simulink model "elevator"  (R2020a)
settings: Solver=VariableStepAuto  StartTime=0.0  StopTime=inf  RelTol=1e-3
PreLoadFcn:
  | slplc.api.loadDataTypes;
undefined symbols (not defined in the file): BOOL, DINT, INT, slplc
libraries: simulink x1
(part 10 of 38)

== system elevator/PLCControllerSuite/__Logic/Task/Program/__Logic/XIC60 ==
  RungIn : Inport  PortDimensions=1
  BlockEnableRead : Subsystem  DisableCoverage=on  TreatAsAtomicUnit=on  mask{PLCLabelTag=_Block_Enable, PLCBlockType=BlockEnableRead}
      mask prompts: PLCLabelTag "Label Tag:"
      mask init:
      | block = gcb;
      | maskObj = Simulink.Mask.get(block);
      | maskObj.Display = sprintf('disp(''%s'');', PLCLabelTag);
      mask Help: web([docroot '/plccoder/ref/blockenableread' '.html']);
      mask DialogControl PLCBlockTitle Prompt: Block Enable Read
      mask Display: disp('_Block_Enable');
  Instruction_Enable : Subsystem  Priority=12  TreatAsAtomicUnit=on
  RungInOverride : Subsystem  DisableCoverage=on  TreatAsAtomicUnit=on
  __CoreVarRead : Subsystem  Tag=CoreVarReadBlock  DisableCoverage=on  TreatAsAtomicUnit=on  mask{PLCBlockType=CoreVarRead}
      mask init:
      | slplc.callbacks.initCoreVariable(gcb, 'read');
      mask Help: web([docroot '/plccoder/ref/__corevarread' '.html']);
      mask DialogControl PLCBlockTitle Prompt: Core Variable Read
  __Format : MATLAB Function  Tag=PLC_Format_Boolean  Priority=20  DisableCoverage=on  InitFcn=slplc.utils.setBlockAppearance('reset', '%<PLCOperandTag>');  StopFcn=slplc.utils.setBlockAppearance('reset', '%<PLCOperandTag>');  TreatAsAtomicUnit=on
  RungOut : Outport  OutDataTypeStr=BOOL  PortDimensions=1  InitialOutput=false  VectorParamsAs1DForOutWhenUnconnected=off
  wires:
  RungIn/1 -> RungInOverride/1(In1)
  Instruction_Enable/1(Rung-condition-out) -> __Format/3(RungOut), RungOut/1
  BlockEnableRead/1(Out1) -> __Format/1(BlockEnable), Instruction_Enable/Enable
  RungInOverride/1(Out1) -> __Format/2(RungIn), Instruction_Enable/1(Rung-condition-in)
  __CoreVarRead/1(y) -> __Format/4(data)  "DataBit"

== system elevator/PLCControllerSuite/__Logic/Task/Program/__Logic/XIC61 ==
  RungIn : Inport  PortDimensions=1
  BlockEnableRead : Subsystem  DisableCoverage=on  TreatAsAtomicUnit=on  mask{PLCLabelTag=_Block_Enable, PLCBlockType=BlockEnableRead}
      mask prompts: PLCLabelTag "Label Tag:"
      mask init:
      | block = gcb;
      | maskObj = Simulink.Mask.get(block);
      | maskObj.Display = sprintf('disp(''%s'');', PLCLabelTag);
      mask Help: web([docroot '/plccoder/ref/blockenableread' '.html']);
      mask DialogControl PLCBlockTitle Prompt: Block Enable Read
      mask Display: disp('_Block_Enable');
  Instruction_Enable : Subsystem  Priority=12  TreatAsAtomicUnit=on
  RungInOverride : Subsystem  DisableCoverage=on  TreatAsAtomicUnit=on
  __CoreVarRead : Subsystem  Tag=CoreVarReadBlock  DisableCoverage=on  TreatAsAtomicUnit=on  mask{PLCBlockType=CoreVarRead}
      mask init:
      | slplc.callbacks.initCoreVariable(gcb, 'read');
      mask Help: web([docroot '/plccoder/ref/__corevarread' '.html']);
      mask DialogControl PLCBlockTitle Prompt: Core Variable Read
  __Format : MATLAB Function  Tag=PLC_Format_Boolean  Priority=20  DisableCoverage=on  InitFcn=slplc.utils.setBlockAppearance('reset', '%<PLCOperandTag>');  StopFcn=slplc.utils.setBlockAppearance('reset', '%<PLCOperandTag>');  TreatAsAtomicUnit=on
  RungOut : Outport  OutDataTypeStr=BOOL  PortDimensions=1  InitialOutput=false  VectorParamsAs1DForOutWhenUnconnected=off
  wires:
  __CoreVarRead/1(y) -> __Format/4(data)  "DataBit"
  RungInOverride/1(Out1) -> Instruction_Enable/1(Rung-condition-in), __Format/2(RungIn)
  BlockEnableRead/1(Out1) -> Instruction_Enable/Enable, __Format/1(BlockEnable)
  Instruction_Enable/1(Rung-condition-out) -> RungOut/1, __Format/3(RungOut)
  RungIn/1 -> RungInOverride/1(In1)

== system elevator/PLCControllerSuite/__Logic/Task/Program/__Logic/XIC62 ==
  RungIn : Inport  PortDimensions=1
  BlockEnableRead : Subsystem  DisableCoverage=on  TreatAsAtomicUnit=on  mask{PLCLabelTag=_Block_Enable, PLCBlockType=BlockEnableRead}
      mask prompts: PLCLabelTag "Label Tag:"
      mask init:
      | block = gcb;
      | maskObj = Simulink.Mask.get(block);
      | maskObj.Display = sprintf('disp(''%s'');', PLCLabelTag);
      mask Help: web([docroot '/plccoder/ref/blockenableread' '.html']);
      mask DialogControl PLCBlockTitle Prompt: Block Enable Read
      mask Display: disp('_Block_Enable');
  Instruction_Enable : Subsystem  Priority=12  TreatAsAtomicUnit=on
  RungInOverride : Subsystem  DisableCoverage=on  TreatAsAtomicUnit=on
  __CoreVarRead : Subsystem  Tag=CoreVarReadBlock  DisableCoverage=on  TreatAsAtomicUnit=on  mask{PLCBlockType=CoreVarRead}
      mask init:
      | slplc.callbacks.initCoreVariable(gcb, 'read');
      mask Help: web([docroot '/plccoder/ref/__corevarread' '.html']);
      mask DialogControl PLCBlockTitle Prompt: Core Variable Read
  __Format : MATLAB Function  Tag=PLC_Format_Boolean  Priority=20  DisableCoverage=on  InitFcn=slplc.utils.setBlockAppearance('reset', '%<PLCOperandTag>');  StopFcn=slplc.utils.setBlockAppearance('reset', '%<PLCOperandTag>');  TreatAsAtomicUnit=on
  RungOut : Outport  OutDataTypeStr=BOOL  PortDimensions=1  InitialOutput=false  VectorParamsAs1DForOutWhenUnconnected=off
  wires:
  __CoreVarRead/1(y) -> __Format/4(data)  "DataBit"
  RungInOverride/1(Out1) -> Instruction_Enable/1(Rung-condition-in), __Format/2(RungIn)
  BlockEnableRead/1(Out1) -> Instruction_Enable/Enable, __Format/1(BlockEnable)
  Instruction_Enable/1(Rung-condition-out) -> RungOut/1, __Format/3(RungOut)
  RungIn/1 -> RungInOverride/1(In1)

== system elevator/PLCControllerSuite/__Logic/Task/Program/__Logic/XIC63 ==
  RungIn : Inport  PortDimensions=1
  BlockEnableRead : Subsystem  DisableCoverage=on  TreatAsAtomicUnit=on  mask{PLCLabelTag=_Block_Enable, PLCBlockType=BlockEnableRead}
      mask prompts: PLCLabelTag "Label Tag:"
      mask init:
      | block = gcb;
      | maskObj = Simulink.Mask.get(block);
      | maskObj.Display = sprintf('disp(''%s'');', PLCLabelTag);
      mask Help: web([docroot '/plccoder/ref/blockenableread' '.html']);
      mask DialogControl PLCBlockTitle Prompt: Block Enable Read
      mask Display: disp('_Block_Enable');
  Instruction_Enable : Subsystem  Priority=12  TreatAsAtomicUnit=on
  RungInOverride : Subsystem  DisableCoverage=on  TreatAsAtomicUnit=on
  __CoreVarRead : Subsystem  Tag=CoreVarReadBlock  DisableCoverage=on  TreatAsAtomicUnit=on  mask{PLCBlockType=CoreVarRead}
      mask init:
      | slplc.callbacks.initCoreVariable(gcb, 'read');
      mask Help: web([docroot '/plccoder/ref/__corevarread' '.html']);
      mask DialogControl PLCBlockTitle Prompt: Core Variable Read
  __Format : MATLAB Function  Tag=PLC_Format_Boolean  Priority=20  DisableCoverage=on  InitFcn=slplc.utils.setBlockAppearance('reset', '%<PLCOperandTag>');  StopFcn=slplc.utils.setBlockAppearance('reset', '%<PLCOperandTag>');  TreatAsAtomicUnit=on
  RungOut : Outport  OutDataTypeStr=BOOL  PortDimensions=1  InitialOutput=false  VectorParamsAs1DForOutWhenUnconnected=off
  wires:
  RungIn/1 -> RungInOverride/1(In1)
  Instruction_Enable/1(Rung-condition-out) -> __Format/3(RungOut), RungOut/1
  BlockEnableRead/1(Out1) -> __Format/1(BlockEnable), Instruction_Enable/Enable
  RungInOverride/1(Out1) -> __Format/2(RungIn), Instruction_Enable/1(Rung-condition-in)
  __CoreVarRead/1(y) -> __Format/4(data)  "DataBit"

== system elevator/PLCControllerSuite/__Logic/Task/Program/__Logic/XIC64 ==
  RungIn : Inport  PortDimensions=1
  BlockEnableRead : Subsystem  DisableCoverage=on  TreatAsAtomicUnit=on  mask{PLCLabelTag=_Block_Enable, PLCBlockType=BlockEnableRead}
      mask prompts: PLCLabelTag "Label Tag:"
      mask init:
      | block = gcb;
      | maskObj = Simulink.Mask.get(block);
      | maskObj.Display = sprintf('disp(''%s'');', PLCLabelTag);
      mask Help: web([docroot '/plccoder/ref/blockenableread' '.html']);
      mask DialogControl PLCBlockTitle Prompt: Block Enable Read
      mask Display: disp('_Block_Enable');
  Instruction_Enable : Subsystem  Priority=12  TreatAsAtomicUnit=on
  RungInOverride : Subsystem  DisableCoverage=on  TreatAsAtomicUnit=on
  __CoreVarRead : Subsystem  Tag=CoreVarReadBlock  DisableCoverage=on  TreatAsAtomicUnit=on  mask{PLCBlockType=CoreVarRead}
      mask init:
      | slplc.callbacks.initCoreVariable(gcb, 'read');
      mask Help: web([docroot '/plccoder/ref/__corevarread' '.html']);
      mask DialogControl PLCBlockTitle Prompt: Core Variable Read
  __Format : MATLAB Function  Tag=PLC_Format_Boolean  Priority=20  DisableCoverage=on  InitFcn=slplc.utils.setBlockAppearance('reset', '%<PLCOperandTag>');  StopFcn=slplc.utils.setBlockAppearance('reset', '%<PLCOperandTag>');  TreatAsAtomicUnit=on
  RungOut : Outport  OutDataTypeStr=BOOL  PortDimensions=1  InitialOutput=false  VectorParamsAs1DForOutWhenUnconnected=off
  wires:
  RungIn/1 -> RungInOverride/1(In1)
  Instruction_Enable/1(Rung-condition-out) -> __Format/3(RungOut), RungOut/1
  BlockEnableRead/1(Out1) -> __Format/1(BlockEnable), Instruction_Enable/Enable
  RungInOverride/1(Out1) -> __Format/2(RungIn), Instruction_Enable/1(Rung-condition-in)
  __CoreVarRead/1(y) -> __Format/4(data)  "DataBit"

== system elevator/PLCControllerSuite/__Logic/Task/Program/__Logic/XIC65 ==
  RungIn : Inport  PortDimensions=1
  BlockEnableRead : Subsystem  DisableCoverage=on  TreatAsAtomicUnit=on  mask{PLCLabelTag=_Block_Enable, PLCBlockType=BlockEnableRead}
      mask prompts: PLCLabelTag "Label Tag:"
      mask init:
      | block = gcb;
      | maskObj = Simulink.Mask.get(block);
      | maskObj.Display = sprintf('disp(''%s'');', PLCLabelTag);
      mask Help: web([docroot '/plccoder/ref/blockenableread' '.html']);
      mask DialogControl PLCBlockTitle Prompt: Block Enable Read
      mask Display: disp('_Block_Enable');
  Instruction_Enable : Subsystem  Priority=12  TreatAsAtomicUnit=on
  RungInOverride : Subsystem  DisableCoverage=on  TreatAsAtomicUnit=on
  __CoreVarRead : Subsystem  Tag=CoreVarReadBlock  DisableCoverage=on  TreatAsAtomicUnit=on  mask{PLCBlockType=CoreVarRead}
      mask init:
      | slplc.callbacks.initCoreVariable(gcb, 'read');
      mask Help: web([docroot '/plccoder/ref/__corevarread' '.html']);
      mask DialogControl PLCBlockTitle Prompt: Core Variable Read
  __Format : MATLAB Function  Tag=PLC_Format_Boolean  Priority=20  DisableCoverage=on  InitFcn=slplc.utils.setBlockAppearance('reset', '%<PLCOperandTag>');  StopFcn=slplc.utils.setBlockAppearance('reset', '%<PLCOperandTag>');  TreatAsAtomicUnit=on
  RungOut : Outport  OutDataTypeStr=BOOL  PortDimensions=1  InitialOutput=false  VectorParamsAs1DForOutWhenUnconnected=off
  wires:
  __CoreVarRead/1(y) -> __Format/4(data)  "DataBit"
  RungInOverride/1(Out1) -> Instruction_Enable/1(Rung-condition-in), __Format/2(RungIn)
  BlockEnableRead/1(Out1) -> Instruction_Enable/Enable, __Format/1(BlockEnable)
  Instruction_Enable/1(Rung-condition-out) -> RungOut/1, __Format/3(RungOut)
  RungIn/1 -> RungInOverride/1(In1)

== system elevator/PLCControllerSuite/__Logic/Task/Program/__Logic/XIC66 ==
  RungIn : Inport  PortDimensions=1
  BlockEnableRead : Subsystem  DisableCoverage=on  TreatAsAtomicUnit=on  mask{PLCLabelTag=_Block_Enable, PLCBlockType=BlockEnableRead}
      mask prompts: PLCLabelTag "Label Tag:"
      mask init:
      | block = gcb;
      | maskObj = Simulink.Mask.get(block);
      | maskObj.Display = sprintf('disp(''%s'');', PLCLabelTag);
      mask Help: web([docroot '/plccoder/ref/blockenableread' '.html']);
      mask DialogControl PLCBlockTitle Prompt: Block Enable Read
      mask Display: disp('_Block_Enable');
  Instruction_Enable : Subsystem  Priority=12  TreatAsAtomicUnit=on
  RungInOverride : Subsystem  DisableCoverage=on  TreatAsAtomicUnit=on
  __CoreVarRead : Subsystem  Tag=CoreVarReadBlock  DisableCoverage=on  TreatAsAtomicUnit=on  mask{PLCBlockType=CoreVarRead}
      mask init:
      | slplc.callbacks.initCoreVariable(gcb, 'read');
      mask Help: web([docroot '/plccoder/ref/__corevarread' '.html']);
      mask DialogControl PLCBlockTitle Prompt: Core Variable Read
  __Format : MATLAB Function  Tag=PLC_Format_Boolean  Priority=20  DisableCoverage=on  InitFcn=slplc.utils.setBlockAppearance('reset', '%<PLCOperandTag>');  StopFcn=slplc.utils.setBlockAppearance('reset', '%<PLCOperandTag>');  TreatAsAtomicUnit=on
  RungOut : Outport  OutDataTypeStr=BOOL  PortDimensions=1  InitialOutput=false  VectorParamsAs1DForOutWhenUnconnected=off
  wires:
  __CoreVarRead/1(y) -> __Format/4(data)  "DataBit"
  RungInOverride/1(Out1) -> Instruction_Enable/1(Rung-condition-in), __Format/2(RungIn)
  BlockEnableRead/1(Out1) -> Instruction_Enable/Enable, __Format/1(BlockEnable)
  Instruction_Enable/1(Rung-condition-out) -> RungOut/1, __Format/3(RungOut)
  RungIn/1 -> RungInOverride/1(In1)

== system elevator/PLCControllerSuite/__Logic/Task/Program/__Logic/XIC67 ==
  RungIn : Inport  PortDimensions=1
  BlockEnableRead : Subsystem  DisableCoverage=on  TreatAsAtomicUnit=on  mask{PLCLabelTag=_Block_Enable, PLCBlockType=BlockEnableRead}
      mask prompts: PLCLabelTag "Label Tag:"
      mask init:
      | block = gcb;
      | maskObj = Simulink.Mask.get(block);
      | maskObj.Display = sprintf('disp(''%s'');', PLCLabelTag);
      mask Help: web([docroot '/plccoder/ref/blockenableread' '.html']);
      mask DialogControl PLCBlockTitle Prompt: Block Enable Read
      mask Display: disp('_Block_Enable');
  Instruction_Enable : Subsystem  Priority=12  TreatAsAtomicUnit=on
  RungInOverride : Subsystem  DisableCoverage=on  TreatAsAtomicUnit=on
  __CoreVarRead : Subsystem  Tag=CoreVarReadBlock  DisableCoverage=on  TreatAsAtomicUnit=on  mask{PLCBlockType=CoreVarRead}
      mask init:
      | slplc.callbacks.initCoreVariable(gcb, 'read');
      mask Help: web([docroot '/plccoder/ref/__corevarread' '.html']);
      mask DialogControl PLCBlockTitle Prompt: Core Variable Read
  __Format : MATLAB Function  Tag=PLC_Format_Boolean  Priority=20  DisableCoverage=on  InitFcn=slplc.utils.setBlockAppearance('reset', '%<PLCOperandTag>');  StopFcn=slplc.utils.setBlockAppearance('reset', '%<PLCOperandTag>');  TreatAsAtomicUnit=on
  RungOut : Outport  OutDataTypeStr=BOOL  PortDimensions=1  InitialOutput=false  VectorParamsAs1DForOutWhenUnconnected=off
  wires:
  RungIn/1 -> RungInOverride/1(In1)
  Instruction_Enable/1(Rung-condition-out) -> __Format/3(RungOut), RungOut/1
  BlockEnableRead/1(Out1) -> __Format/1(BlockEnable), Instruction_Enable/Enable
  RungInOverride/1(Out1) -> __Format/2(RungIn), Instruction_Enable/1(Rung-condition-in)
  __CoreVarRead/1(y) -> __Format/4(data)  "DataBit"

== system elevator/PLCControllerSuite/__Logic/Task/Program/__Logic/XIC68 ==
  RungIn : Inport  PortDimensions=1
  BlockEnableRead : Subsystem  DisableCoverage=on  TreatAsAtomicUnit=on  mask{PLCLabelTag=_Block_Enable, PLCBlockType=BlockEnableRead}
      mask prompts: PLCLabelTag "Label Tag:"
      mask init:
      | block = gcb;
      | maskObj = Simulink.Mask.get(block);
      | maskObj.Display = sprintf('disp(''%s'');', PLCLabelTag);
      mask Help: web([docroot '/plccoder/ref/blockenableread' '.html']);
      mask DialogControl PLCBlockTitle Prompt: Block Enable Read
      mask Display: disp('_Block_Enable');
  Instruction_Enable : Subsystem  Priority=12  TreatAsAtomicUnit=on
  RungInOverride : Subsystem  DisableCoverage=on  TreatAsAtomicUnit=on
  __CoreVarRead : Subsystem  Tag=CoreVarReadBlock  DisableCoverage=on  TreatAsAtomicUnit=on  mask{PLCBlockType=CoreVarRead}
      mask init:
      | slplc.callbacks.initCoreVariable(gcb, 'read');
      mask Help: web([docroot '/plccoder/ref/__corevarread' '.html']);
      mask DialogControl PLCBlockTitle Prompt: Core Variable Read
  __Format : MATLAB Function  Tag=PLC_Format_Boolean  Priority=20  DisableCoverage=on  InitFcn=slplc.utils.setBlockAppearance('reset', '%<PLCOperandTag>');  StopFcn=slplc.utils.setBlockAppearance('reset', '%<PLCOperandTag>');  TreatAsAtomicUnit=on
  RungOut : Outport  OutDataTypeStr=BOOL  PortDimensions=1  InitialOutput=false  VectorParamsAs1DForOutWhenUnconnected=off
  wires:
  __CoreVarRead/1(y) -> __Format/4(data)  "DataBit"
  RungInOverride/1(Out1) -> Instruction_Enable/1(Rung-condition-in), __Format/2(RungIn)
  BlockEnableRead/1(Out1) -> Instruction_Enable/Enable, __Format/1(BlockEnable)
  Instruction_Enable/1(Rung-condition-out) -> RungOut/1, __Format/3(RungOut)
  RungIn/1 -> RungInOverride/1(In1)

== system elevator/PLCControllerSuite/__Logic/Task/Program/__Logic/XIC69 ==
  RungIn : Inport  PortDimensions=1
  BlockEnableRead : Subsystem  DisableCoverage=on  TreatAsAtomicUnit=on  mask{PLCLabelTag=_Block_Enable, PLCBlockType=BlockEnableRead}
      mask prompts: PLCLabelTag "Label Tag:"
      mask init:
      | block = gcb;
      | maskObj = Simulink.Mask.get(block);
      | maskObj.Display = sprintf('disp(''%s'');', PLCLabelTag);
      mask Help: web([docroot '/plccoder/ref/blockenableread' '.html']);
      mask DialogControl PLCBlockTitle Prompt: Block Enable Read
      mask Display: disp('_Block_Enable');
  Instruction_Enable : Subsystem  Priority=12  TreatAsAtomicUnit=on
  RungInOverride : Subsystem  DisableCoverage=on  TreatAsAtomicUnit=on
  __CoreVarRead : Subsystem  Tag=CoreVarReadBlock  DisableCoverage=on  TreatAsAtomicUnit=on  mask{PLCBlockType=CoreVarRead}
      mask init:
      | slplc.callbacks.initCoreVariable(gcb, 'read');
      mask Help: web([docroot '/plccoder/ref/__corevarread' '.html']);
      mask DialogControl PLCBlockTitle Prompt: Core Variable Read
  __Format : MATLAB Function  Tag=PLC_Format_Boolean  Priority=20  DisableCoverage=on  InitFcn=slplc.utils.setBlockAppearance('reset', '%<PLCOperandTag>');  StopFcn=slplc.utils.setBlockAppearance('reset', '%<PLCOperandTag>');  TreatAsAtomicUnit=on
  RungOut : Outport  OutDataTypeStr=BOOL  PortDimensions=1  InitialOutput=false  VectorParamsAs1DForOutWhenUnconnected=off
  wires:
  RungIn/1 -> RungInOverride/1(In1)
  Instruction_Enable/1(Rung-condition-out) -> __Format/3(RungOut), RungOut/1
  BlockEnableRead/1(Out1) -> __Format/1(BlockEnable), Instruction_Enable/Enable
  RungInOverride/1(Out1) -> __Format/2(RungIn), Instruction_Enable/1(Rung-condition-in)
  __CoreVarRead/1(y) -> __Format/4(data)  "DataBit"

== system elevator/PLCControllerSuite/__Logic/Task/Program/__Logic/XIC7 ==
  RungIn : Inport  PortDimensions=1
  BlockEnableRead : Subsystem  DisableCoverage=on  TreatAsAtomicUnit=on  mask{PLCLabelTag=_Block_Enable, PLCBlockType=BlockEnableRead}
      mask prompts: PLCLabelTag "Label Tag:"
      mask init:
      | block = gcb;
      | maskObj = Simulink.Mask.get(block);
      | maskObj.Display = sprintf('disp(''%s'');', PLCLabelTag);
      mask Help: web([docroot '/plccoder/ref/blockenableread' '.html']);
      mask DialogControl PLCBlockTitle Prompt: Block Enable Read
      mask Display: disp('_Block_Enable');
  Instruction_Enable : Subsystem  Priority=12  TreatAsAtomicUnit=on
  RungInOverride : Subsystem  DisableCoverage=on  TreatAsAtomicUnit=on
  __CoreVarRead : Subsystem  Tag=CoreVarReadBlock  DisableCoverage=on  TreatAsAtomicUnit=on  mask{PLCBlockType=CoreVarRead}
      mask init:
      | slplc.callbacks.initCoreVariable(gcb, 'read');
      mask Help: web([docroot '/plccoder/ref/__corevarread' '.html']);
      mask DialogControl PLCBlockTitle Prompt: Core Variable Read
  __Format : MATLAB Function  Tag=PLC_Format_Boolean  Priority=20  DisableCoverage=on  InitFcn=slplc.utils.setBlockAppearance('reset', '%<PLCOperandTag>');  StopFcn=slplc.utils.setBlockAppearance('reset', '%<PLCOperandTag>');  TreatAsAtomicUnit=on
  RungOut : Outport  OutDataTypeStr=BOOL  PortDimensions=1  InitialOutput=false  VectorParamsAs1DForOutWhenUnconnected=off
  wires:
  __CoreVarRead/1(y) -> __Format/4(data)  "DataBit"
  RungInOverride/1(Out1) -> Instruction_Enable/1(Rung-condition-in), __Format/2(RungIn)
  BlockEnableRead/1(Out1) -> Instruction_Enable/Enable, __Format/1(BlockEnable)
  Instruction_Enable/1(Rung-condition-out) -> RungOut/1, __Format/3(RungOut)
  RungIn/1 -> RungInOverride/1(In1)

== system elevator/PLCControllerSuite/__Logic/Task/Program/__Logic/XIC70 ==
  RungIn : Inport  PortDimensions=1
  BlockEnableRead : Subsystem  DisableCoverage=on  TreatAsAtomicUnit=on  mask{PLCLabelTag=_Block_Enable, PLCBlockType=BlockEnableRead}
      mask prompts: PLCLabelTag "Label Tag:"
      mask init:
      | block = gcb;
      | maskObj = Simulink.Mask.get(block);
      | maskObj.Display = sprintf('disp(''%s'');', PLCLabelTag);
      mask Help: web([docroot '/plccoder/ref/blockenableread' '.html']);
      mask DialogControl PLCBlockTitle Prompt: Block Enable Read
      mask Display: disp('_Block_Enable');
  Instruction_Enable : Subsystem  Priority=12  TreatAsAtomicUnit=on
  RungInOverride : Subsystem  DisableCoverage=on  TreatAsAtomicUnit=on
  __CoreVarRead : Subsystem  Tag=CoreVarReadBlock  DisableCoverage=on  TreatAsAtomicUnit=on  mask{PLCBlockType=CoreVarRead}
      mask init:
      | slplc.callbacks.initCoreVariable(gcb, 'read');
      mask Help: web([docroot '/plccoder/ref/__corevarread' '.html']);
      mask DialogControl PLCBlockTitle Prompt: Core Variable Read
  __Format : MATLAB Function  Tag=PLC_Format_Boolean  Priority=20  DisableCoverage=on  InitFcn=slplc.utils.setBlockAppearance('reset', '%<PLCOperandTag>');  StopFcn=slplc.utils.setBlockAppearance('reset', '%<PLCOperandTag>');  TreatAsAtomicUnit=on
  RungOut : Outport  OutDataTypeStr=BOOL  PortDimensions=1  InitialOutput=false  VectorParamsAs1DForOutWhenUnconnected=off
  wires:
  __CoreVarRead/1(y) -> __Format/4(data)  "DataBit"
  RungInOverride/1(Out1) -> Instruction_Enable/1(Rung-condition-in), __Format/2(RungIn)
  BlockEnableRead/1(Out1) -> Instruction_Enable/Enable, __Format/1(BlockEnable)
  Instruction_Enable/1(Rung-condition-out) -> RungOut/1, __Format/3(RungOut)
  RungIn/1 -> RungInOverride/1(In1)

== system elevator/PLCControllerSuite/__Logic/Task/Program/__Logic/XIC71 ==
  RungIn : Inport  PortDimensions=1
  BlockEnableRead : Subsystem  DisableCoverage=on  TreatAsAtomicUnit=on  mask{PLCLabelTag=_Block_Enable, PLCBlockType=BlockEnableRead}
      mask prompts: PLCLabelTag "Label Tag:"
      mask init:
      | block = gcb;
      | maskObj = Simulink.Mask.get(block);
      | maskObj.Display = sprintf('disp(''%s'');', PLCLabelTag);
      mask Help: web([docroot '/plccoder/ref/blockenableread' '.html']);
      mask DialogControl PLCBlockTitle Prompt: Block Enable Read
      mask Display: disp('_Block_Enable');
  Instruction_Enable : Subsystem  Priority=12  TreatAsAtomicUnit=on
  RungInOverride : Subsystem  DisableCoverage=on  TreatAsAtomicUnit=on
  __CoreVarRead : Subsystem  Tag=CoreVarReadBlock  DisableCoverage=on  TreatAsAtomicUnit=on  mask{PLCBlockType=CoreVarRead}
      mask init:
      | slplc.callbacks.initCoreVariable(gcb, 'read');
      mask Help: web([docroot '/plccoder/ref/__corevarread' '.html']);
      mask DialogControl PLCBlockTitle Prompt: Core Variable Read
  __Format : MATLAB Function  Tag=PLC_Format_Boolean  Priority=20  DisableCoverage=on  InitFcn=slplc.utils.setBlockAppearance('reset', '%<PLCOperandTag>');  StopFcn=slplc.utils.setBlockAppearance('reset', '%<PLCOperandTag>');  TreatAsAtomicUnit=on
  RungOut : Outport  OutDataTypeStr=BOOL  PortDimensions=1  InitialOutput=false  VectorParamsAs1DForOutWhenUnconnected=off
  wires:
  __CoreVarRead/1(y) -> __Format/4(data)  "DataBit"
  RungInOverride/1(Out1) -> Instruction_Enable/1(Rung-condition-in), __Format/2(RungIn)
  BlockEnableRead/1(Out1) -> Instruction_Enable/Enable, __Format/1(BlockEnable)
  Instruction_Enable/1(Rung-condition-out) -> RungOut/1, __Format/3(RungOut)
  RungIn/1 -> RungInOverride/1(In1)

== system elevator/PLCControllerSuite/__Logic/Task/Program/__Logic/XIC72 ==
  RungIn : Inport  PortDimensions=1
  BlockEnableRead : Subsystem  DisableCoverage=on  TreatAsAtomicUnit=on  mask{PLCLabelTag=_Block_Enable, PLCBlockType=BlockEnableRead}
      mask prompts: PLCLabelTag "Label Tag:"
      mask init:
      | block = gcb;
      | maskObj = Simulink.Mask.get(block);
      | maskObj.Display = sprintf('disp(''%s'');', PLCLabelTag);
      mask Help: web([docroot '/plccoder/ref/blockenableread' '.html']);
      mask DialogControl PLCBlockTitle Prompt: Block Enable Read
      mask Display: disp('_Block_Enable');
  Instruction_Enable : Subsystem  Priority=12  TreatAsAtomicUnit=on
  RungInOverride : Subsystem  DisableCoverage=on  TreatAsAtomicUnit=on
  __CoreVarRead : Subsystem  Tag=CoreVarReadBlock  DisableCoverage=on  TreatAsAtomicUnit=on  mask{PLCBlockType=CoreVarRead}
      mask init:
      | slplc.callbacks.initCoreVariable(gcb, 'read');
      mask Help: web([docroot '/plccoder/ref/__corevarread' '.html']);
      mask DialogControl PLCBlockTitle Prompt: Core Variable Read
  __Format : MATLAB Function  Tag=PLC_Format_Boolean  Priority=20  DisableCoverage=on  InitFcn=slplc.utils.setBlockAppearance('reset', '%<PLCOperandTag>');  StopFcn=slplc.utils.setBlockAppearance('reset', '%<PLCOperandTag>');  TreatAsAtomicUnit=on
  RungOut : Outport  OutDataTypeStr=BOOL  PortDimensions=1  InitialOutput=false  VectorParamsAs1DForOutWhenUnconnected=off
  wires:
  RungIn/1 -> RungInOverride/1(In1)
  Instruction_Enable/1(Rung-condition-out) -> __Format/3(RungOut), RungOut/1
  BlockEnableRead/1(Out1) -> __Format/1(BlockEnable), Instruction_Enable/Enable
  RungInOverride/1(Out1) -> __Format/2(RungIn), Instruction_Enable/1(Rung-condition-in)
  __CoreVarRead/1(y) -> __Format/4(data)  "DataBit"

== system elevator/PLCControllerSuite/__Logic/Task/Program/__Logic/XIC73 ==
  RungIn : Inport  PortDimensions=1
  BlockEnableRead : Subsystem  DisableCoverage=on  TreatAsAtomicUnit=on  mask{PLCLabelTag=_Block_Enable, PLCBlockType=BlockEnableRead}
      mask prompts: PLCLabelTag "Label Tag:"
      mask init:
      | block = gcb;
      | maskObj = Simulink.Mask.get(block);
      | maskObj.Display = sprintf('disp(''%s'');', PLCLabelTag);
      mask Help: web([docroot '/plccoder/ref/blockenableread' '.html']);
      mask DialogControl PLCBlockTitle Prompt: Block Enable Read
      mask Display: disp('_Block_Enable');
  Instruction_Enable : Subsystem  Priority=12  TreatAsAtomicUnit=on
  RungInOverride : Subsystem  DisableCoverage=on  TreatAsAtomicUnit=on
  __CoreVarRead : Subsystem  Tag=CoreVarReadBlock  DisableCoverage=on  TreatAsAtomicUnit=on  mask{PLCBlockType=CoreVarRead}
      mask init:
      | slplc.callbacks.initCoreVariable(gcb, 'read');
      mask Help: web([docroot '/plccoder/ref/__corevarread' '.html']);
      mask DialogControl PLCBlockTitle Prompt: Core Variable Read
  __Format : MATLAB Function  Tag=PLC_Format_Boolean  Priority=20  DisableCoverage=on  InitFcn=slplc.utils.setBlockAppearance('reset', '%<PLCOperandTag>');  StopFcn=slplc.utils.setBlockAppearance('reset', '%<PLCOperandTag>');  TreatAsAtomicUnit=on
  RungOut : Outport  OutDataTypeStr=BOOL  PortDimensions=1  InitialOutput=false  VectorParamsAs1DForOutWhenUnconnected=off
  wires:
  __CoreVarRead/1(y) -> __Format/4(data)  "DataBit"
  RungInOverride/1(Out1) -> Instruction_Enable/1(Rung-condition-in), __Format/2(RungIn)
  BlockEnableRead/1(Out1) -> Instruction_Enable/Enable, __Format/1(BlockEnable)
  Instruction_Enable/1(Rung-condition-out) -> RungOut/1, __Format/3(RungOut)
  RungIn/1 -> RungInOverride/1(In1)

== system elevator/PLCControllerSuite/__Logic/Task/Program/__Logic/XIC74 ==
  RungIn : Inport  PortDimensions=1
  BlockEnableRead : Subsystem  DisableCoverage=on  TreatAsAtomicUnit=on  mask{PLCLabelTag=_Block_Enable, PLCBlockType=BlockEnableRead}
      mask prompts: PLCLabelTag "Label Tag:"
      mask init:
      | block = gcb;
      | maskObj = Simulink.Mask.get(block);
      | maskObj.Display = sprintf('disp(''%s'');', PLCLabelTag);
      mask Help: web([docroot '/plccoder/ref/blockenableread' '.html']);
      mask DialogControl PLCBlockTitle Prompt: Block Enable Read
      mask Display: disp('_Block_Enable');
  Instruction_Enable : Subsystem  Priority=12  TreatAsAtomicUnit=on
  RungInOverride : Subsystem  DisableCoverage=on  TreatAsAtomicUnit=on
  __CoreVarRead : Subsystem  Tag=CoreVarReadBlock  DisableCoverage=on  TreatAsAtomicUnit=on  mask{PLCBlockType=CoreVarRead}
      mask init:
      | slplc.callbacks.initCoreVariable(gcb, 'read');
      mask Help: web([docroot '/plccoder/ref/__corevarread' '.html']);
      mask DialogControl PLCBlockTitle Prompt: Core Variable Read
  __Format : MATLAB Function  Tag=PLC_Format_Boolean  Priority=20  DisableCoverage=on  InitFcn=slplc.utils.setBlockAppearance('reset', '%<PLCOperandTag>');  StopFcn=slplc.utils.setBlockAppearance('reset', '%<PLCOperandTag>');  TreatAsAtomicUnit=on
  RungOut : Outport  OutDataTypeStr=BOOL  PortDimensions=1  InitialOutput=false  VectorParamsAs1DForOutWhenUnconnected=off
  wires:
  RungIn/1 -> RungInOverride/1(In1)
  Instruction_Enable/1(Rung-condition-out) -> __Format/3(RungOut), RungOut/1
  BlockEnableRead/1(Out1) -> __Format/1(BlockEnable), Instruction_Enable/Enable
  RungInOverride/1(Out1) -> __Format/2(RungIn), Instruction_Enable/1(Rung-condition-in)
  __CoreVarRead/1(y) -> __Format/4(data)  "DataBit"

== system elevator/PLCControllerSuite/__Logic/Task/Program/__Logic/XIC75 ==
  RungIn : Inport  PortDimensions=1
  BlockEnableRead : Subsystem  DisableCoverage=on  TreatAsAtomicUnit=on  mask{PLCLabelTag=_Block_Enable, PLCBlockType=BlockEnableRead}
      mask prompts: PLCLabelTag "Label Tag:"
      mask init:
      | block = gcb;
      | maskObj = Simulink.Mask.get(block);
      | maskObj.Display = sprintf('disp(''%s'');', PLCLabelTag);
      mask Help: web([docroot '/plccoder/ref/blockenableread' '.html']);
      mask DialogControl PLCBlockTitle Prompt: Block Enable Read
      mask Display: disp('_Block_Enable');
  Instruction_Enable : Subsystem  Priority=12  TreatAsAtomicUnit=on
  RungInOverride : Subsystem  DisableCoverage=on  TreatAsAtomicUnit=on
  __CoreVarRead : Subsystem  Tag=CoreVarReadBlock  DisableCoverage=on  TreatAsAtomicUnit=on  mask{PLCBlockType=CoreVarRead}
      mask init:
      | slplc.callbacks.initCoreVariable(gcb, 'read');
      mask Help: web([docroot '/plccoder/ref/__corevarread' '.html']);
      mask DialogControl PLCBlockTitle Prompt: Core Variable Read
  __Format : MATLAB Function  Tag=PLC_Format_Boolean  Priority=20  DisableCoverage=on  InitFcn=slplc.utils.setBlockAppearance('reset', '%<PLCOperandTag>');  StopFcn=slplc.utils.setBlockAppearance('reset', '%<PLCOperandTag>');  TreatAsAtomicUnit=on
  RungOut : Outport  OutDataTypeStr=BOOL  PortDimensions=1  InitialOutput=false  VectorParamsAs1DForOutWhenUnconnected=off
  wires:
  __CoreVarRead/1(y) -> __Format/4(data)  "DataBit"
  RungInOverride/1(Out1) -> Instruction_Enable/1(Rung-condition-in), __Format/2(RungIn)
  BlockEnableRead/1(Out1) -> Instruction_Enable/Enable, __Format/1(BlockEnable)
  Instruction_Enable/1(Rung-condition-out) -> RungOut/1, __Format/3(RungOut)
  RungIn/1 -> RungInOverride/1(In1)

== system elevator/PLCControllerSuite/__Logic/Task/Program/__Logic/XIC76 ==
  RungIn : Inport  PortDimensions=1
  BlockEnableRead : Subsystem  DisableCoverage=on  TreatAsAtomicUnit=on  mask{PLCLabelTag=_Block_Enable, PLCBlockType=BlockEnableRead}
      mask prompts: PLCLabelTag "Label Tag:"
      mask init:
      | block = gcb;
      | maskObj = Simulink.Mask.get(block);
      | maskObj.Display = sprintf('disp(''%s'');', PLCLabelTag);
      mask Help: web([docroot '/plccoder/ref/blockenableread' '.html']);
      mask DialogControl PLCBlockTitle Prompt: Block Enable Read
      mask Display: disp('_Block_Enable');
  Instruction_Enable : Subsystem  Priority=12  TreatAsAtomicUnit=on
  RungInOverride : Subsystem  DisableCoverage=on  TreatAsAtomicUnit=on
  __CoreVarRead : Subsystem  Tag=CoreVarReadBlock  DisableCoverage=on  TreatAsAtomicUnit=on  mask{PLCBlockType=CoreVarRead}
      mask init:
      | slplc.callbacks.initCoreVariable(gcb, 'read');
      mask Help: web([docroot '/plccoder/ref/__corevarread' '.html']);
      mask DialogControl PLCBlockTitle Prompt: Core Variable Read
  __Format : MATLAB Function  Tag=PLC_Format_Boolean  Priority=20  DisableCoverage=on  InitFcn=slplc.utils.setBlockAppearance('reset', '%<PLCOperandTag>');  StopFcn=slplc.utils.setBlockAppearance('reset', '%<PLCOperandTag>');  TreatAsAtomicUnit=on
  RungOut : Outport  OutDataTypeStr=BOOL  PortDimensions=1  InitialOutput=false  VectorParamsAs1DForOutWhenUnconnected=off
  wires:
  RungIn/1 -> RungInOverride/1(In1)
  Instruction_Enable/1(Rung-condition-out) -> __Format/3(RungOut), RungOut/1
  BlockEnableRead/1(Out1) -> __Format/1(BlockEnable), Instruction_Enable/Enable
  RungInOverride/1(Out1) -> __Format/2(RungIn), Instruction_Enable/1(Rung-condition-in)
  __CoreVarRead/1(y) -> __Format/4(data)  "DataBit"

== system elevator/PLCControllerSuite/__Logic/Task/Program/__Logic/XIC77 ==
  RungIn : Inport  PortDimensions=1
  BlockEnableRead : Subsystem  DisableCoverage=on  TreatAsAtomicUnit=on  mask{PLCLabelTag=_Block_Enable, PLCBlockType=BlockEnableRead}
      mask prompts: PLCLabelTag "Label Tag:"
      mask init:
      | block = gcb;
      | maskObj = Simulink.Mask.get(block);
      | maskObj.Display = sprintf('disp(''%s'');', PLCLabelTag);
      mask Help: web([docroot '/plccoder/ref/blockenableread' '.html']);
      mask DialogControl PLCBlockTitle Prompt: Block Enable Read
      mask Display: disp('_Block_Enable');
  Instruction_Enable : Subsystem  Priority=12  TreatAsAtomicUnit=on
  RungInOverride : Subsystem  DisableCoverage=on  TreatAsAtomicUnit=on
  __CoreVarRead : Subsystem  Tag=CoreVarReadBlock  DisableCoverage=on  TreatAsAtomicUnit=on  mask{PLCBlockType=CoreVarRead}
      mask init:
      | slplc.callbacks.initCoreVariable(gcb, 'read');
      mask Help: web([docroot '/plccoder/ref/__corevarread' '.html']);
      mask DialogControl PLCBlockTitle Prompt: Core Variable Read
  __Format : MATLAB Function  Tag=PLC_Format_Boolean  Priority=20  DisableCoverage=on  InitFcn=slplc.utils.setBlockAppearance('reset', '%<PLCOperandTag>');  StopFcn=slplc.utils.setBlockAppearance('reset', '%<PLCOperandTag>');  TreatAsAtomicUnit=on
  RungOut : Outport  OutDataTypeStr=BOOL  PortDimensions=1  InitialOutput=false  VectorParamsAs1DForOutWhenUnconnected=off
  wires:
  RungIn/1 -> RungInOverride/1(In1)
  Instruction_Enable/1(Rung-condition-out) -> __Format/3(RungOut), RungOut/1
  BlockEnableRead/1(Out1) -> __Format/1(BlockEnable), Instruction_Enable/Enable
  RungInOverride/1(Out1) -> __Format/2(RungIn), Instruction_Enable/1(Rung-condition-in)
  __CoreVarRead/1(y) -> __Format/4(data)  "DataBit"

== system elevator/PLCControllerSuite/__Logic/Task/Program/__Logic/XIC78 ==
  RungIn : Inport  PortDimensions=1
  BlockEnableRead : Subsystem  DisableCoverage=on  TreatAsAtomicUnit=on  mask{PLCLabelTag=_Block_Enable, PLCBlockType=BlockEnableRead}
      mask prompts: PLCLabelTag "Label Tag:"
      mask init:
      | block = gcb;
      | maskObj = Simulink.Mask.get(block);
      | maskObj.Display = sprintf('disp(''%s'');', PLCLabelTag);
      mask Help: web([docroot '/plccoder/ref/blockenableread' '.html']);
      mask DialogControl PLCBlockTitle Prompt: Block Enable Read
      mask Display: disp('_Block_Enable');
  Instruction_Enable : Subsystem  Priority=12  TreatAsAtomicUnit=on
  RungInOverride : Subsystem  DisableCoverage=on  TreatAsAtomicUnit=on
  __CoreVarRead : Subsystem  Tag=CoreVarReadBlock  DisableCoverage=on  TreatAsAtomicUnit=on  mask{PLCBlockType=CoreVarRead}
      mask init:
      | slplc.callbacks.initCoreVariable(gcb, 'read');
      mask Help: web([docroot '/plccoder/ref/__corevarread' '.html']);
      mask DialogControl PLCBlockTitle Prompt: Core Variable Read
  __Format : MATLAB Function  Tag=PLC_Format_Boolean  Priority=20  DisableCoverage=on  InitFcn=slplc.utils.setBlockAppearance('reset', '%<PLCOperandTag>');  StopFcn=slplc.utils.setBlockAppearance('reset', '%<PLCOperandTag>');  TreatAsAtomicUnit=on
  RungOut : Outport  OutDataTypeStr=BOOL  PortDimensions=1  InitialOutput=false  VectorParamsAs1DForOutWhenUnconnected=off
  wires:
  RungIn/1 -> RungInOverride/1(In1)
  Instruction_Enable/1(Rung-condition-out) -> __Format/3(RungOut), RungOut/1
  BlockEnableRead/1(Out1) -> __Format/1(BlockEnable), Instruction_Enable/Enable
  RungInOverride/1(Out1) -> __Format/2(RungIn), Instruction_Enable/1(Rung-condition-in)
  __CoreVarRead/1(y) -> __Format/4(data)  "DataBit"

== system elevator/PLCControllerSuite/__Logic/Task/Program/__Logic/XIC79 ==
  RungIn : Inport  PortDimensions=1
  BlockEnableRead : Subsystem  DisableCoverage=on  TreatAsAtomicUnit=on  mask{PLCLabelTag=_Block_Enable, PLCBlockType=BlockEnableRead}
      mask prompts: PLCLabelTag "Label Tag:"
      mask init:
      | block = gcb;
      | maskObj = Simulink.Mask.get(block);
      | maskObj.Display = sprintf('disp(''%s'');', PLCLabelTag);
      mask Help: web([docroot '/plccoder/ref/blockenableread' '.html']);
      mask DialogControl PLCBlockTitle Prompt: Block Enable Read
      mask Display: disp('_Block_Enable');
  Instruction_Enable : Subsystem  Priority=12  TreatAsAtomicUnit=on
  RungInOverride : Subsystem  DisableCoverage=on  TreatAsAtomicUnit=on
  __CoreVarRead : Subsystem  Tag=CoreVarReadBlock  DisableCoverage=on  TreatAsAtomicUnit=on  mask{PLCBlockType=CoreVarRead}
      mask init:
      | slplc.callbacks.initCoreVariable(gcb, 'read');
      mask Help: web([docroot '/plccoder/ref/__corevarread' '.html']);
      mask DialogControl PLCBlockTitle Prompt: Core Variable Read
  __Format : MATLAB Function  Tag=PLC_Format_Boolean  Priority=20  DisableCoverage=on  InitFcn=slplc.utils.setBlockAppearance('reset', '%<PLCOperandTag>');  StopFcn=slplc.utils.setBlockAppearance('reset', '%<PLCOperandTag>');  TreatAsAtomicUnit=on
  RungOut : Outport  OutDataTypeStr=BOOL  PortDimensions=1  InitialOutput=false  VectorParamsAs1DForOutWhenUnconnected=off
  wires:
  __CoreVarRead/1(y) -> __Format/4(data)  "DataBit"
  RungInOverride/1(Out1) -> Instruction_Enable/1(Rung-condition-in), __Format/2(RungIn)
  BlockEnableRead/1(Out1) -> Instruction_Enable/Enable, __Format/1(BlockEnable)
  Instruction_Enable/1(Rung-condition-out) -> RungOut/1, __Format/3(RungOut)
  RungIn/1 -> RungInOverride/1(In1)

== system elevator/PLCControllerSuite/__Logic/Task/Program/__Logic/XIC8 ==
  RungIn : Inport  PortDimensions=1
  BlockEnableRead : Subsystem  DisableCoverage=on  TreatAsAtomicUnit=on  mask{PLCLabelTag=_Block_Enable, PLCBlockType=BlockEnableRead}
      mask prompts: PLCLabelTag "Label Tag:"
      mask init:
      | block = gcb;
      | maskObj = Simulink.Mask.get(block);
      | maskObj.Display = sprintf('disp(''%s'');', PLCLabelTag);
      mask Help: web([docroot '/plccoder/ref/blockenableread' '.html']);
      mask DialogControl PLCBlockTitle Prompt: Block Enable Read
      mask Display: disp('_Block_Enable');
  Instruction_Enable : Subsystem  Priority=12  TreatAsAtomicUnit=on
  RungInOverride : Subsystem  DisableCoverage=on  TreatAsAtomicUnit=on
  __CoreVarRead : Subsystem  Tag=CoreVarReadBlock  DisableCoverage=on  TreatAsAtomicUnit=on  mask{PLCBlockType=CoreVarRead}
      mask init:
      | slplc.callbacks.initCoreVariable(gcb, 'read');
      mask Help: web([docroot '/plccoder/ref/__corevarread' '.html']);
      mask DialogControl PLCBlockTitle Prompt: Core Variable Read
  __Format : MATLAB Function  Tag=PLC_Format_Boolean  Priority=20  DisableCoverage=on  InitFcn=slplc.utils.setBlockAppearance('reset', '%<PLCOperandTag>');  StopFcn=slplc.utils.setBlockAppearance('reset', '%<PLCOperandTag>');  TreatAsAtomicUnit=on
  RungOut : Outport  OutDataTypeStr=BOOL  PortDimensions=1  InitialOutput=false  VectorParamsAs1DForOutWhenUnconnected=off
  wires:
  RungIn/1 -> RungInOverride/1(In1)
  Instruction_Enable/1(Rung-condition-out) -> __Format/3(RungOut), RungOut/1
  BlockEnableRead/1(Out1) -> __Format/1(BlockEnable), Instruction_Enable/Enable
  RungInOverride/1(Out1) -> __Format/2(RungIn), Instruction_Enable/1(Rung-condition-in)
  __CoreVarRead/1(y) -> __Format/4(data)  "DataBit"

== system elevator/PLCControllerSuite/__Logic/Task/Program/__Logic/XIC80 ==
  RungIn : Inport  PortDimensions=1
  BlockEnableRead : Subsystem  DisableCoverage=on  TreatAsAtomicUnit=on  mask{PLCLabelTag=_Block_Enable, PLCBlockType=BlockEnableRead}
      mask prompts: PLCLabelTag "Label Tag:"
      mask init:
      | block = gcb;
      | maskObj = Simulink.Mask.get(block);
      | maskObj.Display = sprintf('disp(''%s'');', PLCLabelTag);
      mask Help: web([docroot '/plccoder/ref/blockenableread' '.html']);
      mask DialogControl PLCBlockTitle Prompt: Block Enable Read
      mask Display: disp('_Block_Enable');
  Instruction_Enable : Subsystem  Priority=12  TreatAsAtomicUnit=on
  RungInOverride : Subsystem  DisableCoverage=on  TreatAsAtomicUnit=on
  __CoreVarRead : Subsystem  Tag=CoreVarReadBlock  DisableCoverage=on  TreatAsAtomicUnit=on  mask{PLCBlockType=CoreVarRead}
      mask init:
      | slplc.callbacks.initCoreVariable(gcb, 'read');
      mask Help: web([docroot '/plccoder/ref/__corevarread' '.html']);
      mask DialogControl PLCBlockTitle Prompt: Core Variable Read
  __Format : MATLAB Function  Tag=PLC_Format_Boolean  Priority=20  DisableCoverage=on  InitFcn=slplc.utils.setBlockAppearance('reset', '%<PLCOperandTag>');  StopFcn=slplc.utils.setBlockAppearance('reset', '%<PLCOperandTag>');  TreatAsAtomicUnit=on
  RungOut : Outport  OutDataTypeStr=BOOL  PortDimensions=1  InitialOutput=false  VectorParamsAs1DForOutWhenUnconnected=off
  wires:
  __CoreVarRead/1(y) -> __Format/4(data)  "DataBit"
  RungInOverride/1(Out1) -> Instruction_Enable/1(Rung-condition-in), __Format/2(RungIn)
  BlockEnableRead/1(Out1) -> Instruction_Enable/Enable, __Format/1(BlockEnable)
  Instruction_Enable/1(Rung-condition-out) -> RungOut/1, __Format/3(RungOut)
  RungIn/1 -> RungInOverride/1(In1)

== system elevator/PLCControllerSuite/__Logic/Task/Program/__Logic/XIC81 ==
  RungIn : Inport  PortDimensions=1
  BlockEnableRead : Subsystem  DisableCoverage=on  TreatAsAtomicUnit=on  mask{PLCLabelTag=_Block_Enable, PLCBlockType=BlockEnableRead}
      mask prompts: PLCLabelTag "Label Tag:"
      mask init:
      | block = gcb;
      | maskObj = Simulink.Mask.get(block);
      | maskObj.Display = sprintf('disp(''%s'');', PLCLabelTag);
      mask Help: web([docroot '/plccoder/ref/blockenableread' '.html']);
      mask DialogControl PLCBlockTitle Prompt: Block Enable Read
      mask Display: disp('_Block_Enable');
  Instruction_Enable : Subsystem  Priority=12  TreatAsAtomicUnit=on
  RungInOverride : Subsystem  DisableCoverage=on  TreatAsAtomicUnit=on
  __CoreVarRead : Subsystem  Tag=CoreVarReadBlock  DisableCoverage=on  TreatAsAtomicUnit=on  mask{PLCBlockType=CoreVarRead}
      mask init:
      | slplc.callbacks.initCoreVariable(gcb, 'read');
      mask Help: web([docroot '/plccoder/ref/__corevarread' '.html']);
      mask DialogControl PLCBlockTitle Prompt: Core Variable Read
  __Format : MATLAB Function  Tag=PLC_Format_Boolean  Priority=20  DisableCoverage=on  InitFcn=slplc.utils.setBlockAppearance('reset', '%<PLCOperandTag>');  StopFcn=slplc.utils.setBlockAppearance('reset', '%<PLCOperandTag>');  TreatAsAtomicUnit=on
  RungOut : Outport  OutDataTypeStr=BOOL  PortDimensions=1  InitialOutput=false  VectorParamsAs1DForOutWhenUnconnected=off
  wires:
  __CoreVarRead/1(y) -> __Format/4(data)  "DataBit"
  RungInOverride/1(Out1) -> Instruction_Enable/1(Rung-condition-in), __Format/2(RungIn)
  BlockEnableRead/1(Out1) -> Instruction_Enable/Enable, __Format/1(BlockEnable)
  Instruction_Enable/1(Rung-condition-out) -> RungOut/1, __Format/3(RungOut)
  RungIn/1 -> RungInOverride/1(In1)

== system elevator/PLCControllerSuite/__Logic/Task/Program/__Logic/XIC82 ==
  RungIn : Inport  PortDimensions=1
  BlockEnableRead : Subsystem  DisableCoverage=on  TreatAsAtomicUnit=on  mask{PLCLabelTag=_Block_Enable, PLCBlockType=BlockEnableRead}
      mask prompts: PLCLabelTag "Label Tag:"
      mask init:
      | block = gcb;
      | maskObj = Simulink.Mask.get(block);
      | maskObj.Display = sprintf('disp(''%s'');', PLCLabelTag);
      mask Help: web([docroot '/plccoder/ref/blockenableread' '.html']);
      mask DialogControl PLCBlockTitle Prompt: Block Enable Read
      mask Display: disp('_Block_Enable');
  Instruction_Enable : Subsystem  Priority=12  TreatAsAtomicUnit=on
  RungInOverride : Subsystem  DisableCoverage=on  TreatAsAtomicUnit=on
  __CoreVarRead : Subsystem  Tag=CoreVarReadBlock  DisableCoverage=on  TreatAsAtomicUnit=on  mask{PLCBlockType=CoreVarRead}
      mask init:
      | slplc.callbacks.initCoreVariable(gcb, 'read');
      mask Help: web([docroot '/plccoder/ref/__corevarread' '.html']);
      mask DialogControl PLCBlockTitle Prompt: Core Variable Read
  __Format : MATLAB Function  Tag=PLC_Format_Boolean  Priority=20  DisableCoverage=on  InitFcn=slplc.utils.setBlockAppearance('reset', '%<PLCOperandTag>');  StopFcn=slplc.utils.setBlockAppearance('reset', '%<PLCOperandTag>');  TreatAsAtomicUnit=on
  RungOut : Outport  OutDataTypeStr=BOOL  PortDimensions=1  InitialOutput=false  VectorParamsAs1DForOutWhenUnconnected=off
  wires:
  RungIn/1 -> RungInOverride/1(In1)
  Instruction_Enable/1(Rung-condition-out) -> __Format/3(RungOut), RungOut/1
  BlockEnableRead/1(Out1) -> __Format/1(BlockEnable), Instruction_Enable/Enable
  RungInOverride/1(Out1) -> __Format/2(RungIn), Instruction_Enable/1(Rung-condition-in)
  __CoreVarRead/1(y) -> __Format/4(data)  "DataBit"

== system elevator/PLCControllerSuite/__Logic/Task/Program/__Logic/XIC83 ==
  RungIn : Inport  PortDimensions=1
  BlockEnableRead : Subsystem  DisableCoverage=on  TreatAsAtomicUnit=on  mask{PLCLabelTag=_Block_Enable, PLCBlockType=BlockEnableRead}
      mask prompts: PLCLabelTag "Label Tag:"
      mask init:
      | block = gcb;
      | maskObj = Simulink.Mask.get(block);
      | maskObj.Display = sprintf('disp(''%s'');', PLCLabelTag);
      mask Help: web([docroot '/plccoder/ref/blockenableread' '.html']);
      mask DialogControl PLCBlockTitle Prompt: Block Enable Read
      mask Display: disp('_Block_Enable');
  Instruction_Enable : Subsystem  Priority=12  TreatAsAtomicUnit=on
  RungInOverride : Subsystem  DisableCoverage=on  TreatAsAtomicUnit=on
  __CoreVarRead : Subsystem  Tag=CoreVarReadBlock  DisableCoverage=on  TreatAsAtomicUnit=on  mask{PLCBlockType=CoreVarRead}
      mask init:
      | slplc.callbacks.initCoreVariable(gcb, 'read');
      mask Help: web([docroot '/plccoder/ref/__corevarread' '.html']);
      mask DialogControl PLCBlockTitle Prompt: Core Variable Read
  __Format : MATLAB Function  Tag=PLC_Format_Boolean  Priority=20  DisableCoverage=on  InitFcn=slplc.utils.setBlockAppearance('reset', '%<PLCOperandTag>');  StopFcn=slplc.utils.setBlockAppearance('reset', '%<PLCOperandTag>');  TreatAsAtomicUnit=on
  RungOut : Outport  OutDataTypeStr=BOOL  PortDimensions=1  InitialOutput=false  VectorParamsAs1DForOutWhenUnconnected=off
  wires:
  RungIn/1 -> RungInOverride/1(In1)
  Instruction_Enable/1(Rung-condition-out) -> __Format/3(RungOut), RungOut/1
  BlockEnableRead/1(Out1) -> __Format/1(BlockEnable), Instruction_Enable/Enable
  RungInOverride/1(Out1) -> __Format/2(RungIn), Instruction_Enable/1(Rung-condition-in)
  __CoreVarRead/1(y) -> __Format/4(data)  "DataBit"

== system elevator/PLCControllerSuite/__Logic/Task/Program/__Logic/XIC84 ==
  RungIn : Inport  PortDimensions=1
  BlockEnableRead : Subsystem  DisableCoverage=on  TreatAsAtomicUnit=on  mask{PLCLabelTag=_Block_Enable, PLCBlockType=BlockEnableRead}
      mask prompts: PLCLabelTag "Label Tag:"
      mask init:
      | block = gcb;
      | maskObj = Simulink.Mask.get(block);
      | maskObj.Display = sprintf('disp(''%s'');', PLCLabelTag);
      mask Help: web([docroot '/plccoder/ref/blockenableread' '.html']);
      mask DialogControl PLCBlockTitle Prompt: Block Enable Read
      mask Display: disp('_Block_Enable');
  Instruction_Enable : Subsystem  Priority=12  TreatAsAtomicUnit=on
  RungInOverride : Subsystem  DisableCoverage=on  TreatAsAtomicUnit=on
  __CoreVarRead : Subsystem  Tag=CoreVarReadBlock  DisableCoverage=on  TreatAsAtomicUnit=on  mask{PLCBlockType=CoreVarRead}
      mask init:
      | slplc.callbacks.initCoreVariable(gcb, 'read');
      mask Help: web([docroot '/plccoder/ref/__corevarread' '.html']);
      mask DialogControl PLCBlockTitle Prompt: Core Variable Read
  __Format : MATLAB Function  Tag=PLC_Format_Boolean  Priority=20  DisableCoverage=on  InitFcn=slplc.utils.setBlockAppearance('reset', '%<PLCOperandTag>');  StopFcn=slplc.utils.setBlockAppearance('reset', '%<PLCOperandTag>');  TreatAsAtomicUnit=on
  RungOut : Outport  OutDataTypeStr=BOOL  PortDimensions=1  InitialOutput=false  VectorParamsAs1DForOutWhenUnconnected=off
  wires:
  __CoreVarRead/1(y) -> __Format/4(data)  "DataBit"
  RungInOverride/1(Out1) -> Instruction_Enable/1(Rung-condition-in), __Format/2(RungIn)
  BlockEnableRead/1(Out1) -> Instruction_Enable/Enable, __Format/1(BlockEnable)
  Instruction_Enable/1(Rung-condition-out) -> RungOut/1, __Format/3(RungOut)
  RungIn/1 -> RungInOverride/1(In1)
